simulink model "IEEE_religador"  (R2021b)
settings: Solver=ode23t  StartTime=0.0  StopTime=4  MaxStep=1e-4  RelTol=1e-3
undefined symbols (not defined in the file or in its folder): D1, Delta
libraries: spsThreePhasePISectionLineLib x36, spsThreePhaseVIMeasurementLib x34, spsSeriesRLCLoadLib x30, dsparch4 x24, spsSampleandHoldLib x24, spsNeutralLib x21, dspstat3 x20, spsPiSectionLineLib x15, spsLoadFlowBusLib x9, spsThreePhaseSeriesRLCLoadLib x8, spsThreePhaseFaultLib x7, spsThreePhaseBreakerLib x5
(part 2 of 2)

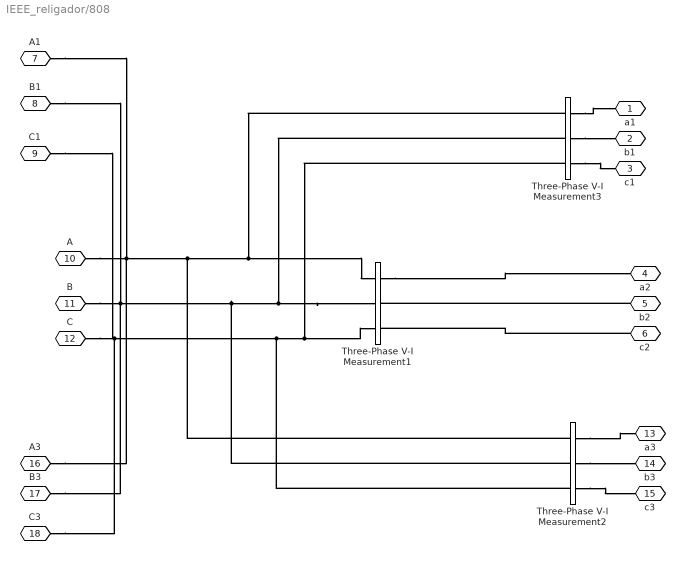
== system IEEE_religador/808 ==
  Three-Phase V-I Measurement1 : spsThreePhaseVIMeasurementLib/Three-Phase V-I Measurement  VoltageMeasurement=phase-to-ground  SetLabelV=on  LabelV=Vabc_3_2  Vpu=off  VpuLL=off  CurrentMeasurement=yes  SetLabelI=on  LabelI=Iabc_3_2  Ipu=off  Pbase=100e6  Vbase=230e3  OutputType=Complex  PhasorSimulation=off  PSBequivalent=0
  Three-Phase V-I Measurement2 : spsThreePhaseVIMeasurementLib/Three-Phase V-I Measurement  VoltageMeasurement=phase-to-ground  SetLabelV=on  LabelV=Vabc_3_3  Vpu=off  VpuLL=off  CurrentMeasurement=yes  SetLabelI=on  LabelI=Iabc_3_3  Ipu=off  Pbase=100e6  Vbase=230e3  OutputType=Complex  PhasorSimulation=off  PSBequivalent=0
  Three-Phase V-I Measurement3 : spsThreePhaseVIMeasurementLib/Three-Phase V-I Measurement  VoltageMeasurement=no  SetLabelV=on  LabelV=Vabc_3_1  Vpu=off  VpuLL=off  CurrentMeasurement=no  SetLabelI=on  LabelI=Iabc_3_1  Ipu=off  Pbase=100e6  Vbase=230e3  OutputType=Complex  PhasorSimulation=off  PSBequivalent=0
  a1 : PMIOPort  Side=Right
  b1 : PMIOPort  Port=2  Side=Right
  c1 : PMIOPort  Port=3  Side=Right
  a2 : PMIOPort  Port=4  Side=Right
  b2 : PMIOPort  Port=5  Side=Right
  c2 : PMIOPort  Port=6  Side=Right
  A1 : PMIOPort  Port=7  Side=Left
  B1 : PMIOPort  Port=8  Side=Left
  C1 : PMIOPort  Port=9  Side=Left
  A : PMIOPort  Port=10  Side=Left
  B : PMIOPort  Port=11  Side=Left
  C : PMIOPort  Port=12  Side=Left
  a3 : PMIOPort  Port=13  Side=Right
  b3 : PMIOPort  Port=14  Side=Right
  c3 : PMIOPort  Port=15  Side=Right
  A3 : PMIOPort  Port=16  Side=Left
  B3 : PMIOPort  Port=17  Side=Left
  C3 : PMIOPort  Port=18  Side=Left
  connections:
  B3/RConn1 -- B1/RConn1 -- Three-Phase V-I Measurement2/LConn2 -- Three-Phase V-I Measurement3/LConn2 -- Three-Phase V-I Measurement1/LConn2 -- B/RConn1
  A/RConn1 -- Three-Phase V-I Measurement2/LConn1 -- Three-Phase V-I Measurement3/LConn1 -- Three-Phase V-I Measurement1/LConn1 -- A3/RConn1 -- A1/RConn1
  C3/RConn1 -- Three-Phase V-I Measurement2/LConn3 -- Three-Phase V-I Measurement3/LConn3 -- Three-Phase V-I Measurement1/LConn3 -- C1/RConn1 -- C/RConn1
  b2/RConn1 -- Three-Phase V-I Measurement1/RConn2
  c2/RConn1 -- Three-Phase V-I Measurement1/RConn3
  Three-Phase V-I Measurement3/RConn1 -- a1/RConn1
  Three-Phase V-I Measurement3/RConn2 -- b1/RConn1
  Three-Phase V-I Measurement3/RConn3 -- c1/RConn1
  Three-Phase V-I Measurement2/RConn1 -- a3/RConn1
  Three-Phase V-I Measurement1/RConn1 -- a2/RConn1
  Three-Phase V-I Measurement2/RConn3 -- c3/RConn1
  Three-Phase V-I Measurement2/RConn2 -- b3/RConn1

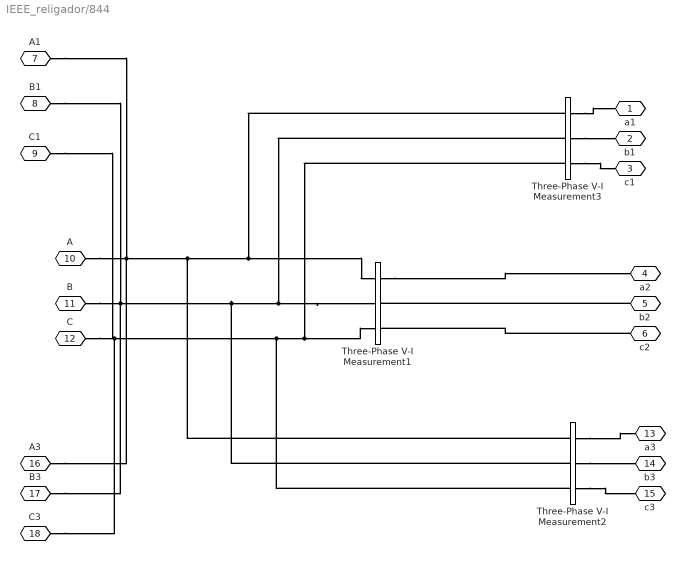
== system IEEE_religador/844 ==
  Three-Phase V-I Measurement1 : spsThreePhaseVIMeasurementLib/Three-Phase V-I Measurement  VoltageMeasurement=no  SetLabelV=on  LabelV=Vabc_3_2  Vpu=off  VpuLL=off  CurrentMeasurement=no  SetLabelI=on  LabelI=Iabc_3_2  Ipu=off  Pbase=100e6  Vbase=230e3  OutputType=Magnitude  PhasorSimulation=off  PSBequivalent=0
  Three-Phase V-I Measurement2 : spsThreePhaseVIMeasurementLib/Three-Phase V-I Measurement  VoltageMeasurement=no  SetLabelV=on  LabelV=Vabc_3_3  Vpu=off  VpuLL=off  CurrentMeasurement=no  SetLabelI=on  LabelI=Iabc_3_3  Ipu=off  Pbase=100e6  Vbase=230e3  OutputType=Complex  PhasorSimulation=off  PSBequivalent=0
  Three-Phase V-I Measurement3 : spsThreePhaseVIMeasurementLib/Three-Phase V-I Measurement  VoltageMeasurement=no  SetLabelV=on  LabelV=Vabc_3_1  Vpu=off  VpuLL=off  CurrentMeasurement=no  SetLabelI=on  LabelI=Iabc_3_1  Ipu=off  Pbase=100e6  Vbase=230e3  OutputType=Complex  PhasorSimulation=off  PSBequivalent=0
  a1 : PMIOPort  Side=Right
  b1 : PMIOPort  Port=2  Side=Right
  c1 : PMIOPort  Port=3  Side=Right
  a2 : PMIOPort  Port=4  Side=Right
  b2 : PMIOPort  Port=5  Side=Right
  c2 : PMIOPort  Port=6  Side=Right
  A1 : PMIOPort  Port=7  Side=Left
  B1 : PMIOPort  Port=8  Side=Left
  C1 : PMIOPort  Port=9  Side=Left
  A : PMIOPort  Port=10  Side=Left
  B : PMIOPort  Port=11  Side=Left
  C : PMIOPort  Port=12  Side=Left
  a3 : PMIOPort  Port=13  Side=Right
  b3 : PMIOPort  Port=14  Side=Right
  c3 : PMIOPort  Port=15  Side=Right
  A3 : PMIOPort  Port=16  Side=Left
  B3 : PMIOPort  Port=17  Side=Left
  C3 : PMIOPort  Port=18  Side=Left
  connections:
  B3/RConn1 -- B1/RConn1 -- Three-Phase V-I Measurement2/LConn2 -- Three-Phase V-I Measurement3/LConn2 -- Three-Phase V-I Measurement1/LConn2 -- B/RConn1
  A/RConn1 -- Three-Phase V-I Measurement2/LConn1 -- Three-Phase V-I Measurement3/LConn1 -- Three-Phase V-I Measurement1/LConn1 -- A3/RConn1 -- A1/RConn1
  C3/RConn1 -- Three-Phase V-I Measurement2/LConn3 -- Three-Phase V-I Measurement3/LConn3 -- Three-Phase V-I Measurement1/LConn3 -- C1/RConn1 -- C/RConn1
  b2/RConn1 -- Three-Phase V-I Measurement1/RConn2
  c2/RConn1 -- Three-Phase V-I Measurement1/RConn3
  Three-Phase V-I Measurement3/RConn1 -- a1/RConn1
  Three-Phase V-I Measurement3/RConn2 -- b1/RConn1
  Three-Phase V-I Measurement3/RConn3 -- c1/RConn1
  Three-Phase V-I Measurement2/RConn1 -- a3/RConn1
  Three-Phase V-I Measurement1/RConn1 -- a2/RConn1
  Three-Phase V-I Measurement2/RConn3 -- c3/RConn1
  Three-Phase V-I Measurement2/RConn2 -- b3/RConn1

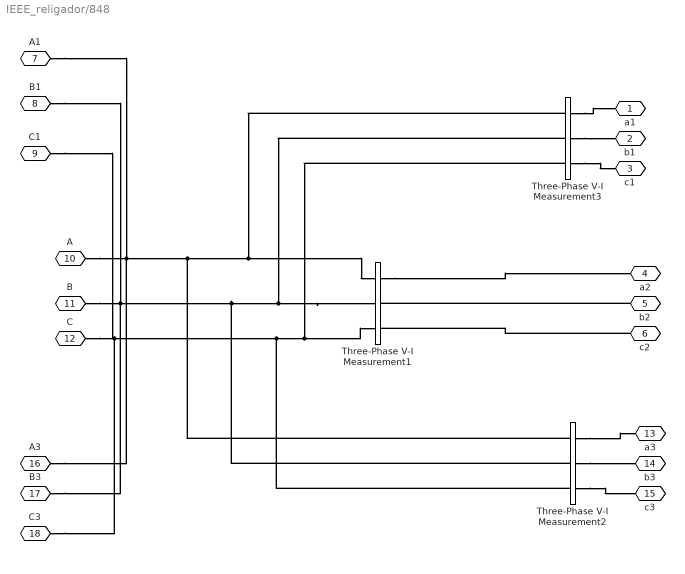
== system IEEE_religador/848 ==
  Three-Phase V-I Measurement1 : spsThreePhaseVIMeasurementLib/Three-Phase V-I Measurement  VoltageMeasurement=no  SetLabelV=on  LabelV=Vabc_3_2  Vpu=off  VpuLL=off  CurrentMeasurement=no  SetLabelI=on  LabelI=Iabc_3_2  Ipu=off  Pbase=100e6  Vbase=230e3  OutputType=Complex  PhasorSimulation=off  PSBequivalent=0
  Three-Phase V-I Measurement2 : spsThreePhaseVIMeasurementLib/Three-Phase V-I Measurement  VoltageMeasurement=no  SetLabelV=on  LabelV=Vabc_3_3  Vpu=off  VpuLL=off  CurrentMeasurement=no  SetLabelI=on  LabelI=Iabc_3_3  Ipu=off  Pbase=100e6  Vbase=230e3  OutputType=Complex  PhasorSimulation=off  PSBequivalent=0
  Three-Phase V-I Measurement3 : spsThreePhaseVIMeasurementLib/Three-Phase V-I Measurement  VoltageMeasurement=no  SetLabelV=on  LabelV=Vabc_848  Vpu=off  VpuLL=off  CurrentMeasurement=no  SetLabelI=on  LabelI=Iabc_848  Ipu=off  Pbase=100e6  Vbase=230e3  OutputType=Complex  PhasorSimulation=off  PSBequivalent=0
  a1 : PMIOPort  Side=Right
  b1 : PMIOPort  Port=2  Side=Right
  c1 : PMIOPort  Port=3  Side=Right
  a2 : PMIOPort  Port=4  Side=Right
  b2 : PMIOPort  Port=5  Side=Right
  c2 : PMIOPort  Port=6  Side=Right
  A1 : PMIOPort  Port=7  Side=Left
  B1 : PMIOPort  Port=8  Side=Left
  C1 : PMIOPort  Port=9  Side=Left
  A : PMIOPort  Port=10  Side=Left
  B : PMIOPort  Port=11  Side=Left
  C : PMIOPort  Port=12  Side=Left
  a3 : PMIOPort  Port=13  Side=Right
  b3 : PMIOPort  Port=14  Side=Right
  c3 : PMIOPort  Port=15  Side=Right
  A3 : PMIOPort  Port=16  Side=Left
  B3 : PMIOPort  Port=17  Side=Left
  C3 : PMIOPort  Port=18  Side=Left
  connections:
  B3/RConn1 -- B1/RConn1 -- Three-Phase V-I Measurement2/LConn2 -- Three-Phase V-I Measurement3/LConn2 -- Three-Phase V-I Measurement1/LConn2 -- B/RConn1
  A/RConn1 -- Three-Phase V-I Measurement2/LConn1 -- Three-Phase V-I Measurement3/LConn1 -- Three-Phase V-I Measurement1/LConn1 -- A3/RConn1 -- A1/RConn1
  C3/RConn1 -- Three-Phase V-I Measurement2/LConn3 -- Three-Phase V-I Measurement3/LConn3 -- Three-Phase V-I Measurement1/LConn3 -- C1/RConn1 -- C/RConn1
  b2/RConn1 -- Three-Phase V-I Measurement1/RConn2
  c2/RConn1 -- Three-Phase V-I Measurement1/RConn3
  Three-Phase V-I Measurement3/RConn1 -- a1/RConn1
  Three-Phase V-I Measurement3/RConn2 -- b1/RConn1
  Three-Phase V-I Measurement3/RConn3 -- c1/RConn1
  Three-Phase V-I Measurement2/RConn1 -- a3/RConn1
  Three-Phase V-I Measurement1/RConn1 -- a2/RConn1
  Three-Phase V-I Measurement2/RConn3 -- c3/RConn1
  Three-Phase V-I Measurement2/RConn2 -- b3/RConn1

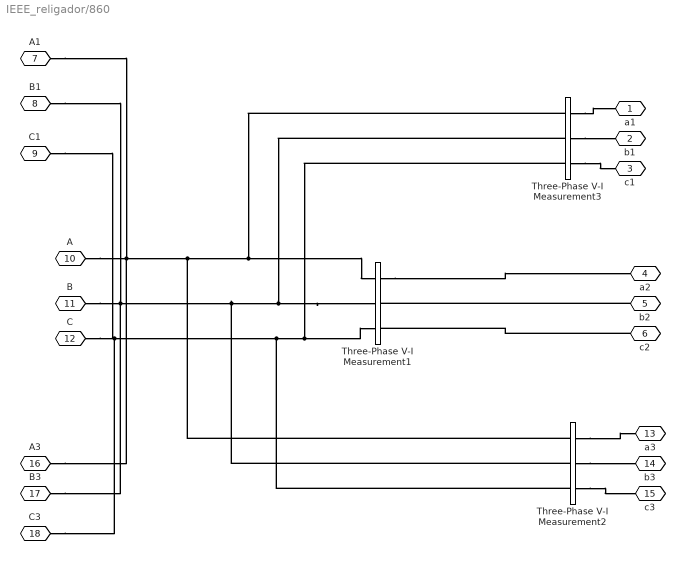
== system IEEE_religador/860 ==
  Three-Phase V-I Measurement1 : spsThreePhaseVIMeasurementLib/Three-Phase V-I Measurement  VoltageMeasurement=no  SetLabelV=on  LabelV=Vabc_3_2  Vpu=off  VpuLL=off  CurrentMeasurement=no  SetLabelI=on  LabelI=Iabc_3_2  Ipu=off  Pbase=100e6  Vbase=230e3  OutputType=Complex  PhasorSimulation=off  PSBequivalent=0
  Three-Phase V-I Measurement2 : spsThreePhaseVIMeasurementLib/Three-Phase V-I Measurement  VoltageMeasurement=no  SetLabelV=on  LabelV=Vabc_3_3  Vpu=off  VpuLL=off  CurrentMeasurement=no  SetLabelI=on  LabelI=Iabc_3_3  Ipu=off  Pbase=100e6  Vbase=230e3  OutputType=Complex  PhasorSimulation=off  PSBequivalent=0
  Three-Phase V-I Measurement3 : spsThreePhaseVIMeasurementLib/Three-Phase V-I Measurement  VoltageMeasurement=no  SetLabelV=on  LabelV=Vabc_3_1  Vpu=off  VpuLL=off  CurrentMeasurement=no  SetLabelI=on  LabelI=Iabc_3_1  Ipu=off  Pbase=100e6  Vbase=230e3  OutputType=Complex  PhasorSimulation=off  PSBequivalent=0
  a1 : PMIOPort  Side=Right
  b1 : PMIOPort  Port=2  Side=Right
  c1 : PMIOPort  Port=3  Side=Right
  a2 : PMIOPort  Port=4  Side=Right
  b2 : PMIOPort  Port=5  Side=Right
  c2 : PMIOPort  Port=6  Side=Right
  A1 : PMIOPort  Port=7  Side=Left
  B1 : PMIOPort  Port=8  Side=Left
  C1 : PMIOPort  Port=9  Side=Left
  A : PMIOPort  Port=10  Side=Left
  B : PMIOPort  Port=11  Side=Left
  C : PMIOPort  Port=12  Side=Left
  a3 : PMIOPort  Port=13  Side=Right
  b3 : PMIOPort  Port=14  Side=Right
  c3 : PMIOPort  Port=15  Side=Right
  A3 : PMIOPort  Port=16  Side=Left
  B3 : PMIOPort  Port=17  Side=Left
  C3 : PMIOPort  Port=18  Side=Left
  connections:
  B3/RConn1 -- B1/RConn1 -- Three-Phase V-I Measurement2/LConn2 -- Three-Phase V-I Measurement3/LConn2 -- Three-Phase V-I Measurement1/LConn2 -- B/RConn1
  A/RConn1 -- Three-Phase V-I Measurement2/LConn1 -- Three-Phase V-I Measurement3/LConn1 -- Three-Phase V-I Measurement1/LConn1 -- A3/RConn1 -- A1/RConn1
  C3/RConn1 -- Three-Phase V-I Measurement2/LConn3 -- Three-Phase V-I Measurement3/LConn3 -- Three-Phase V-I Measurement1/LConn3 -- C1/RConn1 -- C/RConn1
  b2/RConn1 -- Three-Phase V-I Measurement1/RConn2
  c2/RConn1 -- Three-Phase V-I Measurement1/RConn3
  Three-Phase V-I Measurement3/RConn1 -- a1/RConn1
  Three-Phase V-I Measurement3/RConn2 -- b1/RConn1
  Three-Phase V-I Measurement3/RConn3 -- c1/RConn1
  Three-Phase V-I Measurement2/RConn1 -- a3/RConn1
  Three-Phase V-I Measurement1/RConn1 -- a2/RConn1
  Three-Phase V-I Measurement2/RConn3 -- c3/RConn1
  Three-Phase V-I Measurement2/RConn2 -- b3/RConn1

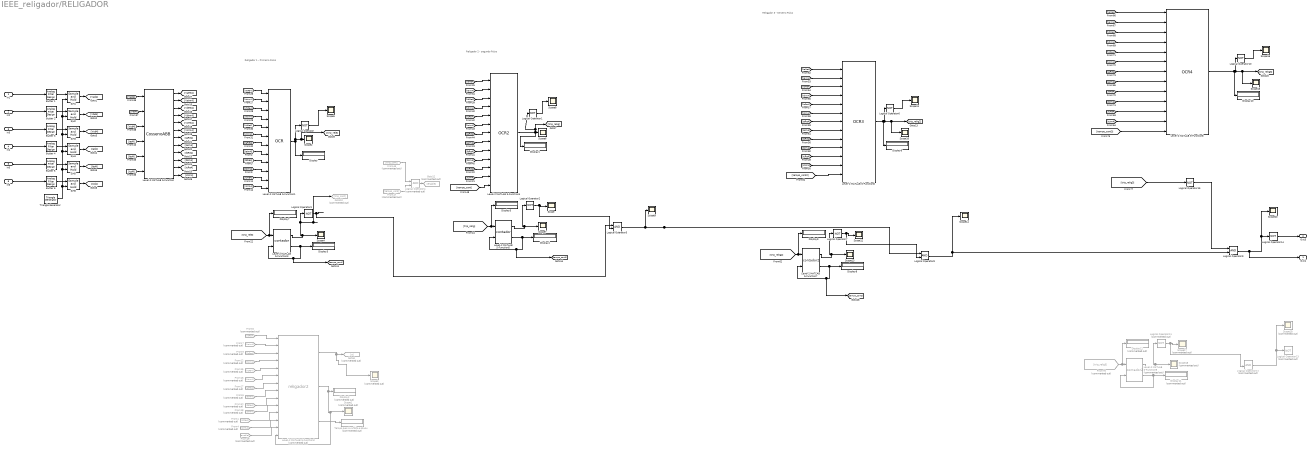
== system IEEE_religador/RELIGADOR ==
  note: Religador 1 - Primeiro Pulso
  note: Religador 2 - segundo Pulso
  note: Religador 3 - terceiro Pulso
  In1 : Inport
  In2 : Inport  Port=2
  In3 : Inport  Port=3
  In4 : Inport  Port=4
  In5 : Inport  Port=5
  In6 : Inport  Port=6
  Butter {1..3,5..6} (5 alike) : dsparch4/Analog Filter Design  method=Butterworth  filttype=Lowpass  N=3  Wlo=2*pi*180  Whi=80  Rp=2  Rs=40
  Butter 4 : dsparch4/Analog Filter Design  method=Butterworth  filttype=Lowpass  N=2  Wlo=6000  Whi=80  Rp=2  Rs=40
  Display{,1,3..10} (10 alike) : Display
  Display11 : Display  Commented=on
  Display12 : Display  Commented=on
  Display2 : Display  Commented=on
  From1 : From  Commented=on  GotoTag=IcRe4
  From12 : From  Commented=on  GotoTag=VbIm4
  From13 : From  Commented=on  GotoTag=IbRe4
  From15 : From  Commented=on  GotoTag=VcRe4
  From16 : From  Commented=on  GotoTag=VcIm4
  From17 : From  Commented=on  GotoTag=IaRe4
  From18 : From  Commented=on  GotoTag=IbIm4
  From19 : From  Commented=on  GotoTag=enable
  From4 : From  Commented=on  GotoTag=IcIm4
  From46 : From  Commented=on  GotoTag=trip_cont
  From47 : From  Commented=on  GotoTag=tempo_cont
  From5 : From  Commented=on  GotoTag=IaIm4
  From6 : From  Commented=on  GotoTag=VaRe4
  From7 : From  Commented=on  GotoTag=VaIm4
  From76 : From  Commented=on  GotoTag=trip_relig3
  From8 : From  Commented=on  GotoTag=VbRe4
  Goto10 : Goto  Commented=on  GotoTag=trip_cont
  Goto12 : Goto  Commented=on  GotoTag=enable
  Goto8 : Goto  Commented=on  GotoTag=a
  Level-2 MATLAB S-Function : M-S-Function  FunctionName=CossenoABB
  Level-2 MATLAB S-Function1 : M-S-Function  FunctionName=OCR  Parameters=Ip, TMS, tau, curvaf, Ipn, TMSn, taun, curvan  mask(S-function: OCR){Ip=56, TMS=0.05, tau=0, curvaf=1, Ipn=16.8, TMSn=0.12, taun=pi/2, curvan=1}
      mask prompts: Ip "Corrente de Pickup (fase)"; TMS "Dial de Tempo (fase)"; tau "Torque (fase)"; curvaf "Tipo de Curva (fase)"; Ipn "Corrente de Pickup (terra)"; TMSn "Dial de Tempo (terra)"; taun "Torque (terra)"; curvan "Tipo de Curva (Terra)"
      mask help: Esta é uma S-Function level-2 que emula um relé de sobrecorrente.
      mask TypeOptions curvaf: 1 | 2 | 3
      mask TypeOptions curvan: 1 | 2 | 3
      mask Display: disp('Relé\nde\nSobrecorrente')
  Level-2 MATLAB S-Function2 : M-S-Function  Commented=on  FunctionName=religador2  Parameters=56,0.05,pi/2,2,16.8,0.12,pi/6,1
  Level-2 MATLAB S-Function3 : M-S-Function  FunctionName=contador
  Level-2 MATLAB S-Function4 : M-S-Function  FunctionName=OCR2  Parameters=56,0.05,0,1,16.8,0.12,pi/2,1
  Level-2 MATLAB S-Function5 : M-S-Function  FunctionName=contador
  Level-2 MATLAB S-Function6 : M-S-Function  FunctionName=OCR3  Parameters=56,0.05,0,1,16.8,0.12,pi/2,1
  Level-2 MATLAB S-Function7 : M-S-Function  FunctionName=contador2
  Level-2 MATLAB S-Function8 : M-S-Function  FunctionName=OCR4  Parameters=56,0.05,0,1,16.8,0.12,pi/2,1
  Level-2 MATLAB S-Function9 : M-S-Function  Commented=on  FunctionName=contador2
  Logical Operator{,1..3,6..7,10,14..15} (9 alike) : Logic  Operator=NOT  AllPortsSameDT=off
  Logical Operator11 : Logic  Commented=on  Operator=NOT  AllPortsSameDT=off
  Logical Operator12 : Logic  Commented=on  AllPortsSameDT=off
  Logical Operator13 : Logic  Commented=on  Operator=NOT  AllPortsSameDT=off
  Logical Operator4 : Logic  Commented=on  AllPortsSameDT=off
  Logical Operator5 : Logic  AllPortsSameDT=off
  Logical Operator8 : Logic  AllPortsSameDT=off
  Logical Operator9 : Logic  AllPortsSameDT=off
  S/H{1..6} (6 alike) : spsSampleandHoldLib/Sample and Hold  ic=0  Ts=1/960
      settings: SourceProductBaseCode=PS
  Scope{,2,4..16,20} (16 alike) : Scope
  Scope{1,3,17..19} (5 alike) : Scope  Commented=on
  Tempo que viu a falta e atuou : Display  Commented=on
  Triangle Generator : spsTriangleGeneratorLib/Triangle Generator  Freq=1/0.00105  Phase=30  Ts=0
  Out1 : Outport  VectorParamsAs1DForOutWhenUnconnected=off
  Out3 : Outport  Port=2  VectorParamsAs1DForOutWhenUnconnected=off
  wires:
  [Ibd4] -> Level-2 MATLAB S-Function/5
  [Vbd4] -> Level-2 MATLAB S-Function/2
  Level-2 MATLAB S-Function/11 -> [IcRe4]
  Level-2 MATLAB S-Function/3 -> [VbRe4]
  Level-2 MATLAB S-Function/5 -> [VcRe4]
  [Vcd4] -> Level-2 MATLAB S-Function/3
  Level-2 MATLAB S-Function/2 -> [VaIm4]
  Level-2 MATLAB S-Function/1 -> [VaRe4]
  Level-2 MATLAB S-Function/4 -> [VbIm4]
  Level-2 MATLAB S-Function/7 -> [IaRe4]
  Level-2 MATLAB S-Function/8 -> [IaIm4]
  [Iad4] -> Level-2 MATLAB S-Function/4
  Level-2 MATLAB S-Function/9 -> [IbRe4]
  Level-2 MATLAB S-Function/10 -> [IbIm4]
  [Icd4] -> Level-2 MATLAB S-Function/6
  Level-2 MATLAB S-Function/6 -> [VcIm4]
  Level-2 MATLAB S-Function/12 -> [IcIm4]
  [Vad4] -> Level-2 MATLAB S-Function/1
  [IcIm4] -> Level-2 MATLAB S-Function1/12
  [VbIm4] -> Level-2 MATLAB S-Function1/4
  [IaRe4] -> Level-2 MATLAB S-Function1/7
  [VaIm4] -> Level-2 MATLAB S-Function1/2
  [VaRe4] -> Level-2 MATLAB S-Function1/1
  [IcRe4] -> Level-2 MATLAB S-Function1/11
  [IbIm4] -> Level-2 MATLAB S-Function1/10
  [VcIm4] -> Level-2 MATLAB S-Function1/6
  [IbRe4] -> Level-2 MATLAB S-Function1/9
  [IaIm4] -> Level-2 MATLAB S-Function1/8
  [VcRe4] -> Level-2 MATLAB S-Function1/5
  [VbRe4] -> Level-2 MATLAB S-Function1/3
  From8/1 -> Level-2 MATLAB S-Function2/3
  From6/1 -> Level-2 MATLAB S-Function2/1
  From7/1 -> Level-2 MATLAB S-Function2/2
  From17/1 -> Level-2 MATLAB S-Function2/7
  From15/1 -> Level-2 MATLAB S-Function2/5
  From16/1 -> Level-2 MATLAB S-Function2/6
  From18/1 -> Level-2 MATLAB S-Function2/10
  From12/1 -> Level-2 MATLAB S-Function2/4
  From4/1 -> Level-2 MATLAB S-Function2/12
  From5/1 -> Level-2 MATLAB S-Function2/8
  From13/1 -> Level-2 MATLAB S-Function2/9
  From1/1 -> Level-2 MATLAB S-Function2/11
  Level-2 MATLAB S-Function2/2 -> Level-2 MATLAB S-Function2/14, Scope1/1, Display2/1
  From19/1 -> Level-2 MATLAB S-Function2/13
  Level-2 MATLAB S-Function2/1 -> Scope3/1, Goto8/1
  Level-2 MATLAB S-Function2/3 -> Tempo que viu a falta e atuou/1
  Level-2 MATLAB S-Function3/1 -> Scope4/1, Goto10/1, Logical Operator3/1
  Logical Operator/1 -> Scope5/1
  Level-2 MATLAB S-Function3/2 -> [tempo_cont], Level-2 MATLAB S-Function3/2, Display3/1
  [trip_rele] -> Display7/1, Level-2 MATLAB S-Function3/1
  Level-2 MATLAB S-Function1/1 -> Logical Operator/1, [trip_rele], Scope2/1, Display/1
  Level-2 MATLAB S-Function5/2 -> [tempo_cont2], Level-2 MATLAB S-Function5/2, Display4/1
  Logical Operator1/1 -> Scope8/1
  [trip_relig] -> Display5/1, Level-2 MATLAB S-Function5/1
  Level-2 MATLAB S-Function5/1 -> Scope7/1, Logical Operator2/1
  [VbRe4] -> Level-2 MATLAB S-Function4/3
  [VaRe4] -> Level-2 MATLAB S-Function4/1
  [VaIm4] -> Level-2 MATLAB S-Function4/2
  [IaRe4] -> Level-2 MATLAB S-Function4/7
  [VcRe4] -> Level-2 MATLAB S-Function4/5
  [VcIm4] -> Level-2 MATLAB S-Function4/6
  [IbIm4] -> Level-2 MATLAB S-Function4/10
  [VbIm4] -> Level-2 MATLAB S-Function4/4
  Level-2 MATLAB S-Function4/1 -> [trip_relig], Logical Operator1/1, Display1/1, Scope6/1
  [IcIm4] -> Level-2 MATLAB S-Function4/12
  Logical Operator2/1 -> Logical Operator5/2, Scope/1
  [IaIm4] -> Level-2 MATLAB S-Function4/8
  [IbRe4] -> Level-2 MATLAB S-Function4/9
  [IcRe4] -> Level-2 MATLAB S-Function4/11
  From46/1 -> Logical Operator4/1
  From47/1 -> Logical Operator4/2
  Logical Operator4/1 -> Goto12/1
  [tempo_cont] -> Level-2 MATLAB S-Function4/13
  Logical Operator3/1 -> Logical Operator5/1
  S/H4/1 -> [Iad4]
  S/H3/1 -> [Vcd4]
  S/H1/1 -> [Vad4]
  Butter 1/1 -> S/H1/1
  In2/1 -> Butter 2/1
  S/H2/1 -> [Vbd4]
  In1/1 -> Butter 1/1
  Butter 5/1 -> S/H5/1
  S/H5/1 -> [Ibd4]
  Butter 6/1 -> S/H6/1
  In3/1 -> Butter 3/1
  In5/1 -> Butter 5/1
  Butter 2/1 -> S/H2/1
  Butter 3/1 -> S/H3/1
  In4/1 -> Butter 4/1
  Triangle Generator/1 -> S/H4/2, S/H1/2, S/H2/2, S/H3/2, S/H5/2, S/H6/2
  In6/1 -> Butter 6/1
  Butter 4/1 -> S/H4/1
  S/H6/1 -> [Icd4]
  Logical Operator5/1 -> Logical Operator8/1, Scope9/1
  [VaRe4] -> Level-2 MATLAB S-Function6/1
  [VaIm4] -> Level-2 MATLAB S-Function6/2
  [VbRe4] -> Level-2 MATLAB S-Function6/3
  [VbIm4] -> Level-2 MATLAB S-Function6/4
  [VcRe4] -> Level-2 MATLAB S-Function6/5
  [VcIm4] -> Level-2 MATLAB S-Function6/6
  [IaRe4] -> Level-2 MATLAB S-Function6/7
  [IaIm4] -> Level-2 MATLAB S-Function6/8
  [IbRe4] -> Level-2 MATLAB S-Function6/9
  [IbIm4] -> Level-2 MATLAB S-Function6/10
  [IcRe4] -> Level-2 MATLAB S-Function6/11
  [IcIm4] -> Level-2 MATLAB S-Function6/12
  [tempo_cont2] -> Level-2 MATLAB S-Function6/13
  Level-2 MATLAB S-Function6/1 -> Display6/1, Logical Operator6/1, Scope10/1, [trip_relig2]
  Logical Operator6/1 -> Scope11/1
  Level-2 MATLAB S-Function7/1 -> Scope13/1, Logical Operator7/1
  Logical Operator7/1 -> Logical Operator8/2, Scope12/1
  [trip_relig2] -> Display9/1, Level-2 MATLAB S-Function7/1
  Level-2 MATLAB S-Function7/2 -> [tempo_cont3], Level-2 MATLAB S-Function7/2, Display8/1
  [VaRe4] -> Level-2 MATLAB S-Function8/1
  [VaIm4] -> Level-2 MATLAB S-Function8/2
  [VbRe4] -> Level-2 MATLAB S-Function8/3
  [VbIm4] -> Level-2 MATLAB S-Function8/4
  [VcRe4] -> Level-2 MATLAB S-Function8/5
  [VcIm4] -> Level-2 MATLAB S-Function8/6
  [IaRe4] -> Level-2 MATLAB S-Function8/7
  [IaIm4] -> Level-2 MATLAB S-Function8/8
  [IbRe4] -> Level-2 MATLAB S-Function8/9
  [IbIm4] -> Level-2 MATLAB S-Function8/10
  [IcRe4] -> Level-2 MATLAB S-Function8/11
  [IcIm4] -> Level-2 MATLAB S-Function8/12
  [tempo_cont3] -> Level-2 MATLAB S-Function8/13
  Level-2 MATLAB S-Function8/1 -> Display10/1, Logical Operator10/1, Scope15/1, [trip_relig3]
  Logical Operator10/1 -> Scope16/1
  From76/1 -> Display12/1, Level-2 MATLAB S-Function9/1
  Logical Operator11/1 -> Logical Operator12/2, Scope17/1
  Level-2 MATLAB S-Function9/2 -> Level-2 MATLAB S-Function9/2, Display11/1
  Logical Operator12/1 -> Scope19/1, Logical Operator13/1
  Level-2 MATLAB S-Function9/1 -> Scope18/1, Logical Operator11/1
  Logical Operator8/1 -> Logical Operator9/2, Scope14/1
  Logical Operator9/1 -> Out1/1, Scope20/1, Logical Operator14/1
  [trip_relig3] -> Logical Operator15/1
  Logical Operator15/1 -> Logical Operator9/1
  Logical Operator14/1 -> Out3/1

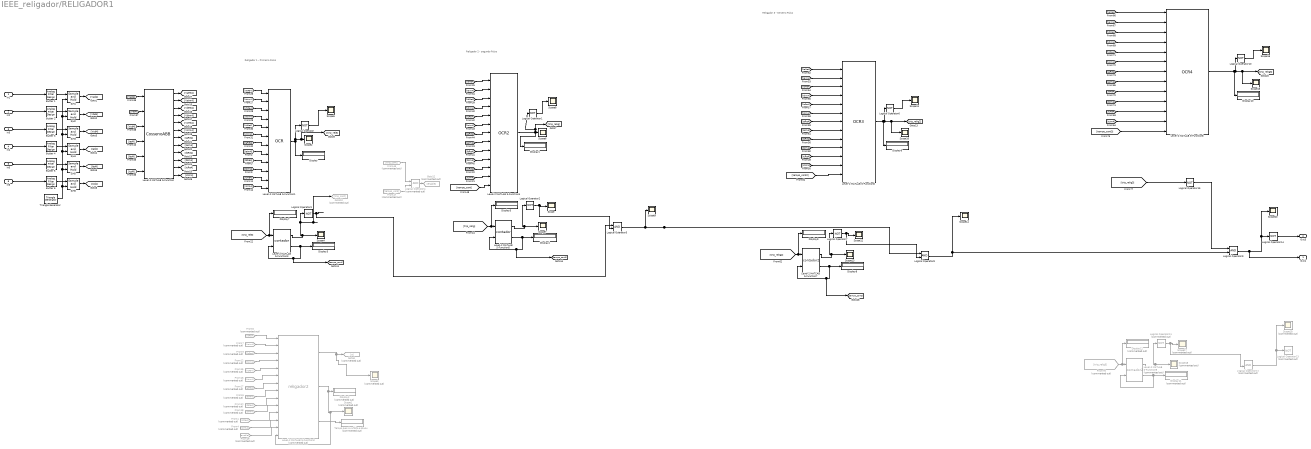
== system IEEE_religador/RELIGADOR1 ==
  note: Religador 1 - Primeiro Pulso
  note: Religador 2 - segundo Pulso
  note: Religador 3 - terceiro Pulso
  In1 : Inport
  In2 : Inport  Port=2
  In3 : Inport  Port=3
  In4 : Inport  Port=4
  In5 : Inport  Port=5
  In6 : Inport  Port=6
  Butter {1..3,5..6} (5 alike) : dsparch4/Analog Filter Design  method=Butterworth  filttype=Lowpass  N=3  Wlo=2*pi*180  Whi=80  Rp=2  Rs=40
  Butter 4 : dsparch4/Analog Filter Design  method=Butterworth  filttype=Lowpass  N=2  Wlo=6000  Whi=80  Rp=2  Rs=40
  Display{,1,3..10} (10 alike) : Display
  Display11 : Display  Commented=on
  Display12 : Display  Commented=on
  Display2 : Display  Commented=on
  From1 : From  Commented=on  GotoTag=IcRe4
  From12 : From  Commented=on  GotoTag=VbIm4
  From13 : From  Commented=on  GotoTag=IbRe4
  From15 : From  Commented=on  GotoTag=VcRe4
  From16 : From  Commented=on  GotoTag=VcIm4
  From17 : From  Commented=on  GotoTag=IaRe4
  From18 : From  Commented=on  GotoTag=IbIm4
  From19 : From  Commented=on  GotoTag=enable
  From4 : From  Commented=on  GotoTag=IcIm4
  From46 : From  Commented=on  GotoTag=trip_cont
  From47 : From  Commented=on  GotoTag=tempo_cont
  From5 : From  Commented=on  GotoTag=IaIm4
  From6 : From  Commented=on  GotoTag=VaRe4
  From7 : From  Commented=on  GotoTag=VaIm4
  From76 : From  Commented=on  GotoTag=trip_relig3
  From8 : From  Commented=on  GotoTag=VbRe4
  Goto10 : Goto  Commented=on  GotoTag=trip_cont
  Goto12 : Goto  Commented=on  GotoTag=enable
  Goto8 : Goto  Commented=on  GotoTag=a
  Level-2 MATLAB S-Function : M-S-Function  FunctionName=CossenoABB
  Level-2 MATLAB S-Function1 : M-S-Function  FunctionName=OCR  Parameters=Ip, TMS, tau, curvaf, Ipn, TMSn, taun, curvan  mask(S-function: OCR){Ip=65, TMS=0.05, tau=0, curvaf=1, Ipn=19, TMSn=0.12, taun=pi/2, curvan=1}
      mask prompts: Ip "Corrente de Pickup (fase)"; TMS "Dial de Tempo (fase)"; tau "Torque (fase)"; curvaf "Tipo de Curva (fase)"; Ipn "Corrente de Pickup (terra)"; TMSn "Dial de Tempo (terra)"; taun "Torque (terra)"; curvan "Tipo de Curva (Terra)"
      mask help: Esta é uma S-Function level-2 que emula um relé de sobrecorrente.
      mask TypeOptions curvaf: 1 | 2 | 3
      mask TypeOptions curvan: 1 | 2 | 3
      mask Display: disp('Relé\nde\nSobrecorrente')
  Level-2 MATLAB S-Function2 : M-S-Function  Commented=on  FunctionName=religador2  Parameters=56,0.05,pi/2,2,16.8,0.12,pi/6,1
  Level-2 MATLAB S-Function3 : M-S-Function  FunctionName=contador
  Level-2 MATLAB S-Function4 : M-S-Function  FunctionName=OCR2  Parameters=65,0.05,0,1,16.8,0.19,pi/2,1
  Level-2 MATLAB S-Function5 : M-S-Function  FunctionName=contador
  Level-2 MATLAB S-Function6 : M-S-Function  FunctionName=OCR3  Parameters=65,0.05,0,1,16.8,0.19,pi/2,1
  Level-2 MATLAB S-Function7 : M-S-Function  FunctionName=contador2
  Level-2 MATLAB S-Function8 : M-S-Function  FunctionName=OCR4  Parameters=65,0.05,0,1,16.8,0.19,pi/2,1
  Level-2 MATLAB S-Function9 : M-S-Function  Commented=on  FunctionName=contador2
  Logical Operator{,1..3,6..7,10,14..15} (9 alike) : Logic  Operator=NOT  AllPortsSameDT=off
  Logical Operator11 : Logic  Commented=on  Operator=NOT  AllPortsSameDT=off
  Logical Operator12 : Logic  Commented=on  AllPortsSameDT=off
  Logical Operator13 : Logic  Commented=on  Operator=NOT  AllPortsSameDT=off
  Logical Operator4 : Logic  Commented=on  AllPortsSameDT=off
  Logical Operator5 : Logic  AllPortsSameDT=off
  Logical Operator8 : Logic  AllPortsSameDT=off
  Logical Operator9 : Logic  AllPortsSameDT=off
  S/H{1..6} (6 alike) : spsSampleandHoldLib/Sample and Hold  ic=0  Ts=1/960
      settings: SourceProductBaseCode=PS
  Scope{,2,4..16,20} (16 alike) : Scope
  Scope{1,3,17..19} (5 alike) : Scope  Commented=on
  Tempo que viu a falta e atuou : Display  Commented=on
  Triangle Generator : spsTriangleGeneratorLib/Triangle Generator  Freq=1/0.00105  Phase=30  Ts=0
  Out1 : Outport  VectorParamsAs1DForOutWhenUnconnected=off
  Out3 : Outport  Port=2  VectorParamsAs1DForOutWhenUnconnected=off
  wires:
  [Ibd4] -> Level-2 MATLAB S-Function/5
  [Vbd4] -> Level-2 MATLAB S-Function/2
  Level-2 MATLAB S-Function/11 -> [IcRe4]
  Level-2 MATLAB S-Function/3 -> [VbRe4]
  Level-2 MATLAB S-Function/5 -> [VcRe4]
  [Vcd4] -> Level-2 MATLAB S-Function/3
  Level-2 MATLAB S-Function/2 -> [VaIm4]
  Level-2 MATLAB S-Function/1 -> [VaRe4]
  Level-2 MATLAB S-Function/4 -> [VbIm4]
  Level-2 MATLAB S-Function/7 -> [IaRe4]
  Level-2 MATLAB S-Function/8 -> [IaIm4]
  [Iad4] -> Level-2 MATLAB S-Function/4
  Level-2 MATLAB S-Function/9 -> [IbRe4]
  Level-2 MATLAB S-Function/10 -> [IbIm4]
  [Icd4] -> Level-2 MATLAB S-Function/6
  Level-2 MATLAB S-Function/6 -> [VcIm4]
  Level-2 MATLAB S-Function/12 -> [IcIm4]
  [Vad4] -> Level-2 MATLAB S-Function/1
  [IcIm4] -> Level-2 MATLAB S-Function1/12
  [VbIm4] -> Level-2 MATLAB S-Function1/4
  [IaRe4] -> Level-2 MATLAB S-Function1/7
  [VaIm4] -> Level-2 MATLAB S-Function1/2
  [VaRe4] -> Level-2 MATLAB S-Function1/1
  [IcRe4] -> Level-2 MATLAB S-Function1/11
  [IbIm4] -> Level-2 MATLAB S-Function1/10
  [VcIm4] -> Level-2 MATLAB S-Function1/6
  [IbRe4] -> Level-2 MATLAB S-Function1/9
  [IaIm4] -> Level-2 MATLAB S-Function1/8
  [VcRe4] -> Level-2 MATLAB S-Function1/5
  [VbRe4] -> Level-2 MATLAB S-Function1/3
  From8/1 -> Level-2 MATLAB S-Function2/3
  From6/1 -> Level-2 MATLAB S-Function2/1
  From7/1 -> Level-2 MATLAB S-Function2/2
  From17/1 -> Level-2 MATLAB S-Function2/7
  From15/1 -> Level-2 MATLAB S-Function2/5
  From16/1 -> Level-2 MATLAB S-Function2/6
  From18/1 -> Level-2 MATLAB S-Function2/10
  From12/1 -> Level-2 MATLAB S-Function2/4
  From4/1 -> Level-2 MATLAB S-Function2/12
  From5/1 -> Level-2 MATLAB S-Function2/8
  From13/1 -> Level-2 MATLAB S-Function2/9
  From1/1 -> Level-2 MATLAB S-Function2/11
  Level-2 MATLAB S-Function2/2 -> Level-2 MATLAB S-Function2/14, Scope1/1, Display2/1
  From19/1 -> Level-2 MATLAB S-Function2/13
  Level-2 MATLAB S-Function2/1 -> Scope3/1, Goto8/1
  Level-2 MATLAB S-Function2/3 -> Tempo que viu a falta e atuou/1
  Level-2 MATLAB S-Function3/1 -> Scope4/1, Goto10/1, Logical Operator3/1
  Logical Operator/1 -> Scope5/1
  Level-2 MATLAB S-Function3/2 -> [tempo_cont], Level-2 MATLAB S-Function3/2, Display3/1
  [trip_rele] -> Display7/1, Level-2 MATLAB S-Function3/1
  Level-2 MATLAB S-Function1/1 -> Logical Operator/1, [trip_rele], Scope2/1, Display/1
  Level-2 MATLAB S-Function5/2 -> [tempo_cont2], Level-2 MATLAB S-Function5/2, Display4/1
  Logical Operator1/1 -> Scope8/1
  [trip_relig] -> Display5/1, Level-2 MATLAB S-Function5/1
  Level-2 MATLAB S-Function5/1 -> Scope7/1, Logical Operator2/1
  [VbRe4] -> Level-2 MATLAB S-Function4/3
  [VaRe4] -> Level-2 MATLAB S-Function4/1
  [VaIm4] -> Level-2 MATLAB S-Function4/2
  [IaRe4] -> Level-2 MATLAB S-Function4/7
  [VcRe4] -> Level-2 MATLAB S-Function4/5
  [VcIm4] -> Level-2 MATLAB S-Function4/6
  [IbIm4] -> Level-2 MATLAB S-Function4/10
  [VbIm4] -> Level-2 MATLAB S-Function4/4
  Level-2 MATLAB S-Function4/1 -> [trip_relig], Logical Operator1/1, Display1/1, Scope6/1
  [IcIm4] -> Level-2 MATLAB S-Function4/12
  Logical Operator2/1 -> Logical Operator5/2, Scope/1
  [IaIm4] -> Level-2 MATLAB S-Function4/8
  [IbRe4] -> Level-2 MATLAB S-Function4/9
  [IcRe4] -> Level-2 MATLAB S-Function4/11
  From46/1 -> Logical Operator4/1
  From47/1 -> Logical Operator4/2
  Logical Operator4/1 -> Goto12/1
  [tempo_cont] -> Level-2 MATLAB S-Function4/13
  Logical Operator3/1 -> Logical Operator5/1
  S/H4/1 -> [Iad4]
  S/H3/1 -> [Vcd4]
  S/H1/1 -> [Vad4]
  Butter 1/1 -> S/H1/1
  In2/1 -> Butter 2/1
  S/H2/1 -> [Vbd4]
  In1/1 -> Butter 1/1
  Butter 5/1 -> S/H5/1
  S/H5/1 -> [Ibd4]
  Butter 6/1 -> S/H6/1
  In3/1 -> Butter 3/1
  In5/1 -> Butter 5/1
  Butter 2/1 -> S/H2/1
  Butter 3/1 -> S/H3/1
  In4/1 -> Butter 4/1
  Triangle Generator/1 -> S/H4/2, S/H1/2, S/H2/2, S/H3/2, S/H5/2, S/H6/2
  In6/1 -> Butter 6/1
  Butter 4/1 -> S/H4/1
  S/H6/1 -> [Icd4]
  Logical Operator5/1 -> Logical Operator8/1, Scope9/1
  [VaRe4] -> Level-2 MATLAB S-Function6/1
  [VaIm4] -> Level-2 MATLAB S-Function6/2
  [VbRe4] -> Level-2 MATLAB S-Function6/3
  [VbIm4] -> Level-2 MATLAB S-Function6/4
  [VcRe4] -> Level-2 MATLAB S-Function6/5
  [VcIm4] -> Level-2 MATLAB S-Function6/6
  [IaRe4] -> Level-2 MATLAB S-Function6/7
  [IaIm4] -> Level-2 MATLAB S-Function6/8
  [IbRe4] -> Level-2 MATLAB S-Function6/9
  [IbIm4] -> Level-2 MATLAB S-Function6/10
  [IcRe4] -> Level-2 MATLAB S-Function6/11
  [IcIm4] -> Level-2 MATLAB S-Function6/12
  [tempo_cont2] -> Level-2 MATLAB S-Function6/13
  Level-2 MATLAB S-Function6/1 -> Display6/1, Logical Operator6/1, Scope10/1, [trip_relig2]
  Logical Operator6/1 -> Scope11/1
  Level-2 MATLAB S-Function7/1 -> Scope13/1, Logical Operator7/1
  Logical Operator7/1 -> Logical Operator8/2, Scope12/1
  [trip_relig2] -> Display9/1, Level-2 MATLAB S-Function7/1
  Level-2 MATLAB S-Function7/2 -> [tempo_cont3], Level-2 MATLAB S-Function7/2, Display8/1
  [VaRe4] -> Level-2 MATLAB S-Function8/1
  [VaIm4] -> Level-2 MATLAB S-Function8/2
  [VbRe4] -> Level-2 MATLAB S-Function8/3
  [VbIm4] -> Level-2 MATLAB S-Function8/4
  [VcRe4] -> Level-2 MATLAB S-Function8/5
  [VcIm4] -> Level-2 MATLAB S-Function8/6
  [IaRe4] -> Level-2 MATLAB S-Function8/7
  [IaIm4] -> Level-2 MATLAB S-Function8/8
  [IbRe4] -> Level-2 MATLAB S-Function8/9
  [IbIm4] -> Level-2 MATLAB S-Function8/10
  [IcRe4] -> Level-2 MATLAB S-Function8/11
  [IcIm4] -> Level-2 MATLAB S-Function8/12
  [tempo_cont3] -> Level-2 MATLAB S-Function8/13
  Level-2 MATLAB S-Function8/1 -> Display10/1, Logical Operator10/1, Scope15/1, [trip_relig3]
  Logical Operator10/1 -> Scope16/1
  From76/1 -> Display12/1, Level-2 MATLAB S-Function9/1
  Logical Operator11/1 -> Logical Operator12/2, Scope17/1
  Level-2 MATLAB S-Function9/2 -> Level-2 MATLAB S-Function9/2, Display11/1
  Logical Operator12/1 -> Scope19/1, Logical Operator13/1
  Level-2 MATLAB S-Function9/1 -> Scope18/1, Logical Operator11/1
  Logical Operator8/1 -> Logical Operator9/2, Scope14/1
  Logical Operator9/1 -> Out1/1, Scope20/1, Logical Operator14/1
  [trip_relig3] -> Logical Operator15/1
  Logical Operator15/1 -> Logical Operator9/1
  Logical Operator14/1 -> Out3/1

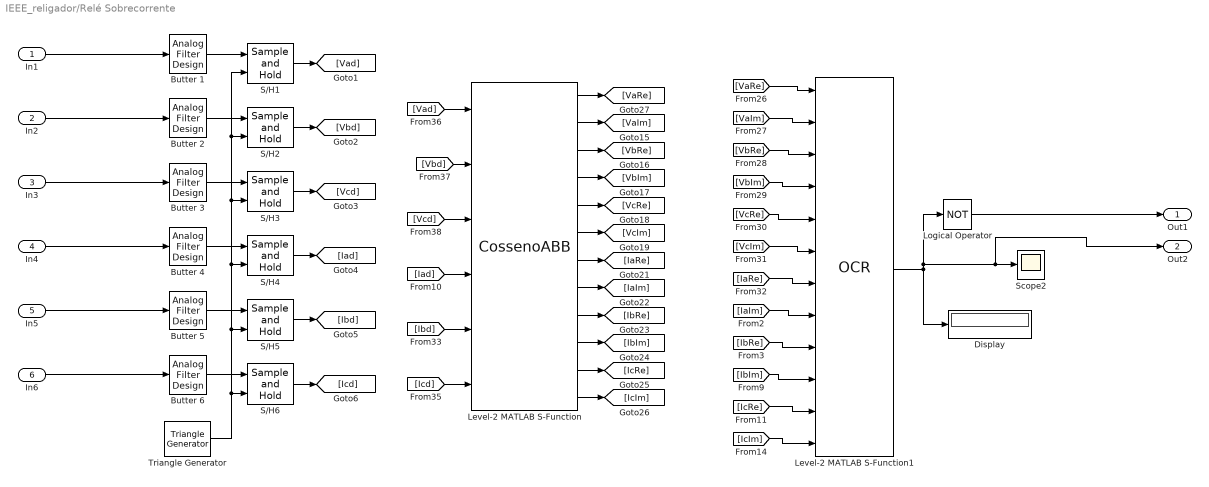
== system IEEE_religador/Relé Sobrecorrente ==
  In1 : Inport
  In2 : Inport  Port=2
  In3 : Inport  Port=3
  In4 : Inport  Port=4
  In5 : Inport  Port=5
  In6 : Inport  Port=6
  Butter {1..3,5..6} (5 alike) : dsparch4/Analog Filter Design  method=Butterworth  filttype=Lowpass  N=3  Wlo=2*pi*180  Whi=80  Rp=2  Rs=40
  Butter 4 : dsparch4/Analog Filter Design  method=Butterworth  filttype=Lowpass  N=2  Wlo=6000  Whi=80  Rp=2  Rs=40
  Display : Display
  Level-2 MATLAB S-Function : M-S-Function  FunctionName=CossenoABB
  Level-2 MATLAB S-Function1 : M-S-Function  FunctionName=OCR  Parameters=Ip, TMS, tau, curvaf, Ipn, TMSn, taun, curvan  mask(S-function: OCR){Ip=75.5, TMS=0.12, tau=pi/6, curvaf=3, Ipn=22.7, TMSn=0.56, taun=pi/6, curvan=2}
      mask prompts: Ip "Corrente de Pickup (fase)"; TMS "Dial de Tempo (fase)"; tau "Torque (fase)"; curvaf "Tipo de Curva (fase)"; Ipn "Corrente de Pickup (terra)"; TMSn "Dial de Tempo (terra)"; taun "Torque (terra)"; curvan "Tipo de Curva (Terra)"
      mask help: Esta é uma S-Function level-2 que emula um relé de sobrecorrente.
      mask TypeOptions curvaf: 1 | 2 | 3
      mask TypeOptions curvan: 1 | 2 | 3
      mask Display: disp('Relé\nde\nSobrecorrente')
  Logical Operator : Logic  Operator=NOT  AllPortsSameDT=off
  S/H{1..6} (6 alike) : spsSampleandHoldLib/Sample and Hold  ic=0  Ts=1/960
      settings: SourceProductBaseCode=PS
  Scope2 : Scope
  Triangle Generator : spsTriangleGeneratorLib/Triangle Generator  Freq=1/0.00105  Phase=30  Ts=0
  Out1 : Outport  VectorParamsAs1DForOutWhenUnconnected=off
  Out2 : Outport  Port=2  VectorParamsAs1DForOutWhenUnconnected=off
  wires:
  [Ibd] -> Level-2 MATLAB S-Function/5
  S/H3/1 -> [Vcd]
  Triangle Generator/1 -> S/H4/2, S/H1/2, S/H2/2, S/H3/2, S/H5/2, S/H6/2
  [Vbd] -> Level-2 MATLAB S-Function/2
  S/H2/1 -> [Vbd]
  Butter 2/1 -> S/H2/1
  S/H1/1 -> [Vad]
  In6/1 -> Butter 6/1
  In3/1 -> Butter 3/1
  In4/1 -> Butter 4/1
  Level-2 MATLAB S-Function/11 -> [IcRe]
  Level-2 MATLAB S-Function/3 -> [VbRe]
  S/H5/1 -> [Ibd]
  Level-2 MATLAB S-Function/5 -> [VcRe]
  [Vcd] -> Level-2 MATLAB S-Function/3
  Level-2 MATLAB S-Function/2 -> [VaIm]
  Level-2 MATLAB S-Function/1 -> [VaRe]
  Level-2 MATLAB S-Function/4 -> [VbIm]
  Butter 6/1 -> S/H6/1
  In5/1 -> Butter 5/1
  Butter 3/1 -> S/H3/1
  In1/1 -> Butter 1/1
  Butter 5/1 -> S/H5/1
  Level-2 MATLAB S-Function/7 -> [IaRe]
  Level-2 MATLAB S-Function/8 -> [IaIm]
  [Iad] -> Level-2 MATLAB S-Function/4
  Butter 1/1 -> S/H1/1
  Level-2 MATLAB S-Function/9 -> [IbRe]
  Level-2 MATLAB S-Function/10 -> [IbIm]
  [Icd] -> Level-2 MATLAB S-Function/6
  Level-2 MATLAB S-Function/6 -> [VcIm]
  In2/1 -> Butter 2/1
  Level-2 MATLAB S-Function/12 -> [IcIm]
  S/H6/1 -> [Icd]
  [Vad] -> Level-2 MATLAB S-Function/1
  [IcIm] -> Level-2 MATLAB S-Function1/12
  [VbIm] -> Level-2 MATLAB S-Function1/4
  [IaRe] -> Level-2 MATLAB S-Function1/7
  [VaIm] -> Level-2 MATLAB S-Function1/2
  [VaRe] -> Level-2 MATLAB S-Function1/1
  Logical Operator/1 -> Out1/1
  [IcRe] -> Level-2 MATLAB S-Function1/11
  [IbIm] -> Level-2 MATLAB S-Function1/10
  [VcIm] -> Level-2 MATLAB S-Function1/6
  [IbRe] -> Level-2 MATLAB S-Function1/9
  [IaIm] -> Level-2 MATLAB S-Function1/8
  Level-2 MATLAB S-Function1/1 -> Logical Operator/1, Out2/1, Scope2/1, Display/1
  [VcRe] -> Level-2 MATLAB S-Function1/5
  [VbRe] -> Level-2 MATLAB S-Function1/3
  S/H4/1 -> [Iad]
  Butter 4/1 -> S/H4/1

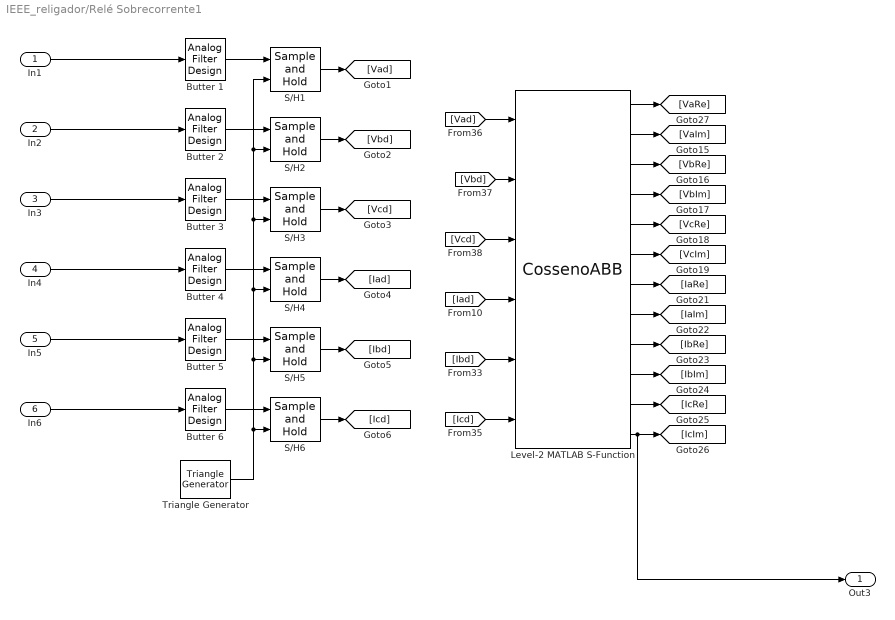
== system IEEE_religador/Relé Sobrecorrente1 ==
  In1 : Inport
  In2 : Inport  Port=2
  In3 : Inport  Port=3
  In4 : Inport  Port=4
  In5 : Inport  Port=5
  In6 : Inport  Port=6
  Butter {1..3,5..6} (5 alike) : dsparch4/Analog Filter Design  method=Butterworth  filttype=Lowpass  N=3  Wlo=2*pi*180  Whi=80  Rp=2  Rs=40
  Butter 4 : dsparch4/Analog Filter Design  method=Butterworth  filttype=Lowpass  N=2  Wlo=6000  Whi=80  Rp=2  Rs=40
  Level-2 MATLAB S-Function : M-S-Function  FunctionName=CossenoABB
  S/H{1..6} (6 alike) : spsSampleandHoldLib/Sample and Hold  ic=0  Ts=1/960
      settings: SourceProductBaseCode=PS
  Triangle Generator : spsTriangleGeneratorLib/Triangle Generator  Freq=1/0.00105  Phase=30  Ts=0
  Out3 : Outport  VectorParamsAs1DForOutWhenUnconnected=off
  wires:
  [Ibd] -> Level-2 MATLAB S-Function/5
  S/H3/1 -> [Vcd]
  Triangle Generator/1 -> S/H4/2, S/H1/2, S/H2/2, S/H3/2, S/H5/2, S/H6/2
  [Vbd] -> Level-2 MATLAB S-Function/2
  S/H2/1 -> [Vbd]
  Butter 2/1 -> S/H2/1
  S/H1/1 -> [Vad]
  In6/1 -> Butter 6/1
  In3/1 -> Butter 3/1
  In4/1 -> Butter 4/1
  Level-2 MATLAB S-Function/11 -> [IcRe]
  Level-2 MATLAB S-Function/3 -> [VbRe]
  S/H5/1 -> [Ibd]
  Level-2 MATLAB S-Function/5 -> [VcRe]
  [Vcd] -> Level-2 MATLAB S-Function/3
  Level-2 MATLAB S-Function/2 -> [VaIm]
  Level-2 MATLAB S-Function/1 -> [VaRe]
  Level-2 MATLAB S-Function/4 -> [VbIm]
  Butter 6/1 -> S/H6/1
  In5/1 -> Butter 5/1
  Butter 3/1 -> S/H3/1
  In1/1 -> Butter 1/1
  Butter 5/1 -> S/H5/1
  Level-2 MATLAB S-Function/7 -> [IaRe]
  Level-2 MATLAB S-Function/8 -> [IaIm]
  [Iad] -> Level-2 MATLAB S-Function/4
  Butter 1/1 -> S/H1/1
  Level-2 MATLAB S-Function/9 -> [IbRe]
  Level-2 MATLAB S-Function/10 -> [IbIm]
  [Icd] -> Level-2 MATLAB S-Function/6
  Level-2 MATLAB S-Function/6 -> [VcIm]
  In2/1 -> Butter 2/1
  S/H6/1 -> [Icd]
  [Vad] -> Level-2 MATLAB S-Function/1
  S/H4/1 -> [Iad]
  Butter 4/1 -> S/H4/1
  Level-2 MATLAB S-Function/12 -> Out3/1, [IcIm]
